simulink model "No6_QuadcopterTrackPositionControl"  (R2022a)
settings: Solver=FixedStepDiscrete  StartTime=0.0  StopTime=Inf  RelTol=1e-3  EnableMultiTasking=on
undefined symbols (not defined in the file): dev, DiscIntNeverNeededParam, Main, pwm_output0
libraries: slpidlib x7, simulink x1, px4lib x1, px4uORBlib x1, sharedtransform x1
settings Model: PacingRate=1000  ExtModeTrigDuration=10  Creator=liuwhale  LastModifiedBy=liuwhale
settings SolverCC: PositivePriorityOrder=on
settings DataIOCC: ReturnWorkspaceOutputsName=tp3ab4fdac_68ba_4606_82f6_9556b5dbcc17
settings OptimizationCC: EnhancedBackFolding=on  PassReuseOutputArgsAs=Individual arguments  ZeroExternalMemoryAtStartup=off  ZeroInternalMemoryAtStartup=off  MaxStackSize=64  OptimizeBlockOrder=speed  DifferentSizesBufferReuse=on  EfficientTunableParamExpr=on
settings DebuggingCC: ParameterTunabilityLossMsg=error
settings HardwareCC: ProdBitPerPointer=32  ProdBitPerSizeT=32  ProdBitPerPtrDiffT=32  ProdLargestAtomicInteger=Long  ProdLargestAtomicFloat=Double  ProdWordSize=32  ProdLongLongMode=on  ProdHWDeviceType=ARM Compatible->ARM Cortex
settings SFSimCC: MATLABDynamicMemAlloc=off  SimTargetLang=C++
settings RTWCC: SystemTargetFile=ert.tlc  HardwareBoard=PX4 Host Target  TLCOptions="-aInlineSetEventsForThisBaseRateFcn=TLC_FALSE -aSuppressMultiTaskScheduler=TLC_FALSE  -aRateBasedStepFcn=0"  TemplateMakefile=ert_default_tmf  Toolchain=GNU Tools for PX4 Autopilots  PortableWordSizes=on  TargetLang=C++
settings CodeAppCC: ForceParamTrailComments=on  IgnoreCustomStorageClasses=off  OperatorAnnotations=on  SimulinkDataObjDesc=on  SFDataObjDesc=on  InsertBlockDesc=on
settings ERTTargetCC: ExtModeStaticAlloc=on

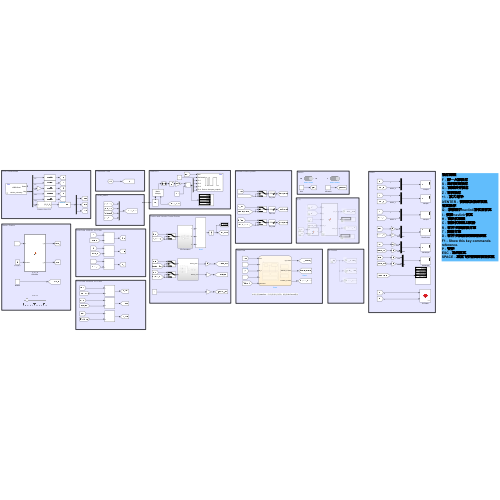
[thumbnail: Simulink's stored preview of the top-level diagram]
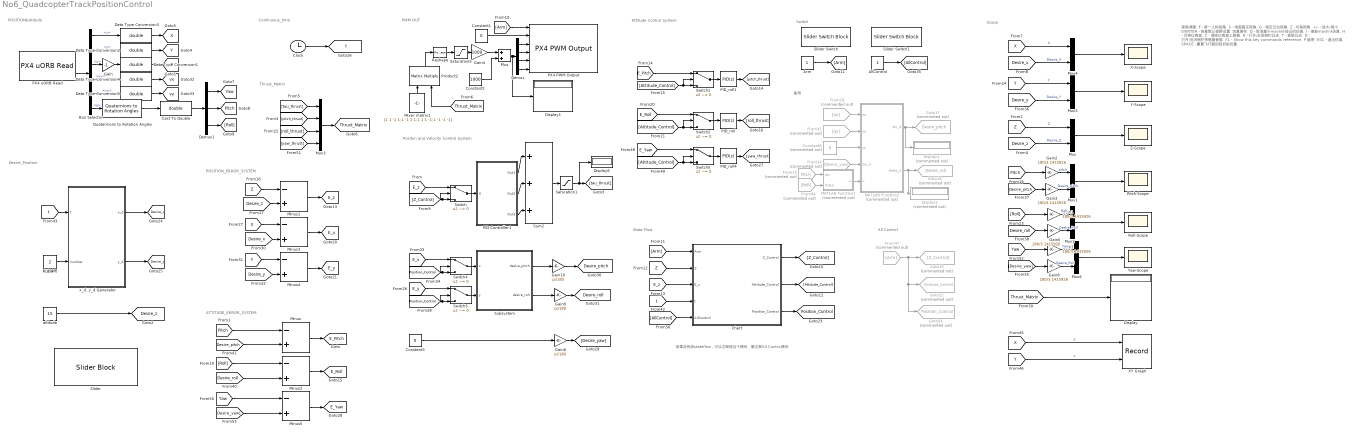
== system No6_QuadcopterTrackPositionControl ==
  note: 如果没有装stateflow，可以注释掉这个模块，解注释All Control模块
  note: All Control
  note: Desire_Position
  note: 备用
  note: 视角调整:
      | F - 第一人称视角.
      | S - 地面固定视角.
      | G - 稳定云台视角.
      | Z - 切换视角.
      | +/- - 放大/缩小
      | 0/ENTER - 恢复默认视野设置.
      | 仿真操作:
      | Q - 取消基于mavlink协议的仿真.
      | I - 使能mavlink仿真.
      | H - 切换仪表盘.
      | C - 清除仪表盘上数据.
      | R - 打开/关闭侧栏日志.
      | T - 更新日志.
      | D - 打开/关闭侧栏传感器参数.
      | F1 - Show this key commands reference.
      | P - 暂停.
      | ESC - 退出仿真.
      | SPACE - 重置飞行器回到初始位置.
  note: State Flow
  note: PWM OUT
  note: Scope
  note: Positon and Velocity Control System
  note: Thrust_Matrix
  note: POSITION_ERROR_SYSTEM
  note: POSITION&Atitude
  note: Continuous_time
  note: Switch
  note: Attitude Control System
  note: ATTITUDE_ERROR_SYSTEM
  AllControl : Constant  OutDataTypeStr=boolean
  Arm : Constant  OutDataTypeStr=boolean
  Bus Selector : BusSelector  OutputSignals=x,y,z,vx,vy,q
  Cast To Double : DataTypeConversion  OutDataTypeStr=double  SaturateOnIntegerOverflow=off  RndMeth=Floor
  Chart : Stateflow chart  TreatAsAtomicUnit=on
  Clock : Clock
  Constant1 : Constant  Value=0  OutDataTypeStr=boolean
  Constant2 : Constant  Value=1000  OutDataTypeStr=uint16
  Constant3 : Constant  Value=0
  Constant6 : Constant  Commented=on  Value=0
  Data Type Conversion{1..5} (5 alike) : DataTypeConversion  OutDataTypeStr=double  SaturateOnIntegerOverflow=off  RndMeth=Floor
  Demux : Demux
  Demux1 : Demux  Outputs=3
  Display : Display
  Display1 : Display
  Display4 : Display  Commented=on
  Display5 : Display  Commented=on
  Display6 : Display
  From25 : From  Commented=on  GotoTag=Pitch  TagVisibility=global
  From29 : From  Commented=on  GotoTag=qx
  From35 : From  Commented=on  GotoTag=qy
  From44 : From  Commented=on  GotoTag=Roll
  From47 : From  Commented=on  GotoTag=Arm
  From54 : From  Commented=on  GotoTag=Desire_yaw
  Gain : Gain  Gain=-1
  Gain{1..3,5,7..8} (6 alike) : Gain  Gain=180/3.1415926
  Gain10 : Gain  Gain=pi/180
  Gain4 : Gain  Gain=1000  OutDataTypeStr=uint16
  Gain6 : Gain  Gain=pi/180
  Gain9 : Gain  Gain=pi/180
  Goto17 : Goto  Commented=on  GotoTag=Desire_pitch  TagVisibility=global
  Goto18 : Goto  Commented=on  GotoTag=Desire_roll  TagVisibility=global
  Goto19 : Goto  Commented=on  GotoTag=Z_Control
  Goto22 : Goto  Commented=on  GotoTag=Attitude_Control
  Goto34 : Goto  Commented=on  GotoTag=Position_Control  TagVisibility=global
  MATLAB Function1 : MATLAB Function  Commented=on  TreatAsAtomicUnit=on
  MATLAB Function2 : MATLAB Function  Commented=on  TreatAsAtomicUnit=on
  Minus{,1..5} (6 alike) : Sum  Inputs=-+
  Mixer matrix1 : Constant  Value=[1 1 -1 1;1 -1 1 1;1 1 1 -1;1 -1 -1 -1]  OutDataTypeStr=Inherit: Inherit via back propagation
  Mux{,1..2,4..6} (6 alike) : Mux  Inputs=2
  Mux3 : Mux
  PID Controller1 : Subsystem
  PID_roll : slpidlib/PID Controller  Controller=PID  Form=Parallel  TimeDomain=Discrete-time  UseExternalTs=off  SampleTime=-1  IntegratorMethod=Backward Euler  FilterMethod=Forward Euler  ControllerParametersSource=internal  P=0.038  I=0.06  UseKiTs=off  D=0.001  N=100  UseFilter=on  TunerSelectOption=Transfer Function Based (PID Tuner App)  InitialConditionSource=internal  InitialConditionForIntegrator=0  InitialConditionForFilter=0  DifferentiatorICPrevScaledInput=0  ExternalReset=none  TrackingMode=off  Kt=1  LimitOutput=on  SatLimitsSource=internal  UpperSaturationLimit=0.01  LowerSaturationLimit=-0.01  LinearizeAsGain=off  AntiWindupMode=none  Kb=1  POutMin=[]  POutMax=[]  IOutMin=[]  IOutMax=[]  DOutMin=[]  DOutMax=[]  NOutMin=[]  NOutMax=[]  SumOutMin=[]  SumOutMax=[]  SaturationOutMin=[]  SaturationOutMax=[]  PParamMin=[]  PParamMax=[]  IParamMin=[]  IParamMax=[]  DParamMin=[]  DParamMax=[]  NParamMin=[]  NParamMax=[]  KbParamMin=[]  KbParamMax=[]  KtParamMin=[]  KtParamMax=[]  KbOutMin=[]  KbOutMax=[]  KtOutMin=[]  KtOutMax=[]  IntegratorOutMin=[]  IntegratorOutMax=[]  FilterOutMin=[]  FilterOutMax=[]  SumI1OutMin=[]  SumI1OutMax=[]  SumI2OutMin=[]  SumI2OutMax=[]  SumI3OutMin=[]  SumI3OutMax=[]  SumI4OutMin=[]  SumI4OutMax=[]  SumDOutMin=[]  SumDOutMax=[]  DifferentiatorOutMin=[]  DifferentiatorOutMax=[]  FilterDiffOutCoefMin=[]  FilterDiffOutCoefMax=[]  ReciprocalOutMin=[]  ReciprocalOutMax=[]  SumDenOutMin=[]  SumDenOutMax=[]  SumNumOutMin=[]  SumNumOutMax=[]  DivideOutMin=[]  DivideOutMax=[]  UdiffTsProdOutMin=[]  UdiffTsProdOutMax=[]  NTsProdOutMin=[]  NTsProdOutMax=[]  UintegralTsProdOutMin=[]  UintegralTsProdOutMax=[]  UngainTsProdOutMin=[]  UngainTsProdOutMax=[]  IntegratorContinuousStateAttributes=''  IntegratorStateMustResolveToSignalObject=off  IntegratorRTWStateStorageClass=Auto  FilterContinuousStateAttributes=''  FilterStateMustResolveToSignalObject=off  FilterRTWStateStorageClass=Auto  ParallelPVariant=InternalParameters  IdealPVariant=Disabled  IVariant=InternalParameters  DVariant=InternalParameters  IntegratorVariant=Discrete  SatVariant=Enabled  AWVariant=Passthrough  PCopyVariant=Disabled  TRVariant=Disabled  FdbkBlocksVariant=Forward  IdealPFdbkVariant=Disabled  SatFdbkVariant=Disabled  DerivativeFilterVariant=ForwardEulerFilter  NVariant=InternalParameters  NCopyVariant=Disabled  FilterICVariant=InternalICsFilter  IntegratorICVariant=InternalICs  ExternalResetVariant=Disabled  TRSumVariant=Passthrough  SumFdbkVariant=Disabled  SumVariant=Sum_PID  TsampFilterVariant=InternalTs  TsampNgainVariant=Passthrough  TsampIntegralVariant=Passthrough  ExternalSaturationOutDataTypeStr=Inherit: Same as second input  aMode=0
  PID_roll1 : slpidlib/PID Controller  Controller=PID  Form=Parallel  TimeDomain=Discrete-time  UseExternalTs=off  SampleTime=-1  IntegratorMethod=Backward Euler  FilterMethod=Forward Euler  ControllerParametersSource=internal  P=0.038  I=0.06  UseKiTs=off  D=0.001  N=100  UseFilter=on  TunerSelectOption=Transfer Function Based (PID Tuner App)  InitialConditionSource=internal  InitialConditionForIntegrator=0  InitialConditionForFilter=0  DifferentiatorICPrevScaledInput=0  ExternalReset=none  TrackingMode=off  Kt=1  LimitOutput=on  SatLimitsSource=internal  UpperSaturationLimit=0.01  LowerSaturationLimit=-0.01  LinearizeAsGain=off  AntiWindupMode=none  Kb=1  POutMin=[]  POutMax=[]  IOutMin=[]  IOutMax=[]  DOutMin=[]  DOutMax=[]  NOutMin=[]  NOutMax=[]  SumOutMin=[]  SumOutMax=[]  SaturationOutMin=[]  SaturationOutMax=[]  PParamMin=[]  PParamMax=[]  IParamMin=[]  IParamMax=[]  DParamMin=[]  DParamMax=[]  NParamMin=[]  NParamMax=[]  KbParamMin=[]  KbParamMax=[]  KtParamMin=[]  KtParamMax=[]  KbOutMin=[]  KbOutMax=[]  KtOutMin=[]  KtOutMax=[]  IntegratorOutMin=[]  IntegratorOutMax=[]  FilterOutMin=[]  FilterOutMax=[]  SumI1OutMin=[]  SumI1OutMax=[]  SumI2OutMin=[]  SumI2OutMax=[]  SumI3OutMin=[]  SumI3OutMax=[]  SumI4OutMin=[]  SumI4OutMax=[]  SumDOutMin=[]  SumDOutMax=[]  DifferentiatorOutMin=[]  DifferentiatorOutMax=[]  FilterDiffOutCoefMin=[]  FilterDiffOutCoefMax=[]  ReciprocalOutMin=[]  ReciprocalOutMax=[]  SumDenOutMin=[]  SumDenOutMax=[]  SumNumOutMin=[]  SumNumOutMax=[]  DivideOutMin=[]  DivideOutMax=[]  UdiffTsProdOutMin=[]  UdiffTsProdOutMax=[]  NTsProdOutMin=[]  NTsProdOutMax=[]  UintegralTsProdOutMin=[]  UintegralTsProdOutMax=[]  UngainTsProdOutMin=[]  UngainTsProdOutMax=[]  IntegratorContinuousStateAttributes=''  IntegratorStateMustResolveToSignalObject=off  IntegratorRTWStateStorageClass=Auto  FilterContinuousStateAttributes=''  FilterStateMustResolveToSignalObject=off  FilterRTWStateStorageClass=Auto  ParallelPVariant=InternalParameters  IdealPVariant=Disabled  IVariant=InternalParameters  DVariant=InternalParameters  IntegratorVariant=Discrete  SatVariant=Enabled  AWVariant=Passthrough  PCopyVariant=Disabled  TRVariant=Disabled  FdbkBlocksVariant=Forward  IdealPFdbkVariant=Disabled  SatFdbkVariant=Disabled  DerivativeFilterVariant=ForwardEulerFilter  NVariant=InternalParameters  NCopyVariant=Disabled  FilterICVariant=InternalICsFilter  IntegratorICVariant=InternalICs  ExternalResetVariant=Disabled  TRSumVariant=Passthrough  SumFdbkVariant=Disabled  SumVariant=Sum_PID  TsampFilterVariant=InternalTs  TsampNgainVariant=Passthrough  TsampIntegralVariant=Passthrough  ExternalSaturationOutDataTypeStr=Inherit: Same as second input  aMode=0
  PID_roll4 : slpidlib/PID Controller  Controller=PID  Form=Parallel  TimeDomain=Discrete-time  UseExternalTs=off  SampleTime=-1  IntegratorMethod=Backward Euler  FilterMethod=Forward Euler  ControllerParametersSource=internal  P=0.055  I=0.05  UseKiTs=off  D=0.003  N=100  UseFilter=on  TunerSelectOption=Transfer Function Based (PID Tuner App)  InitialConditionSource=internal  InitialConditionForIntegrator=0  InitialConditionForFilter=0  DifferentiatorICPrevScaledInput=0  ExternalReset=none  TrackingMode=off  Kt=1  LimitOutput=on  SatLimitsSource=internal  UpperSaturationLimit=0.01  LowerSaturationLimit=-0.01  LinearizeAsGain=off  AntiWindupMode=none  Kb=1  POutMin=[]  POutMax=[]  IOutMin=[]  IOutMax=[]  DOutMin=[]  DOutMax=[]  NOutMin=[]  NOutMax=[]  SumOutMin=[]  SumOutMax=[]  SaturationOutMin=[]  SaturationOutMax=[]  PParamMin=[]  PParamMax=[]  IParamMin=[]  IParamMax=[]  DParamMin=[]  DParamMax=[]  NParamMin=[]  NParamMax=[]  KbParamMin=[]  KbParamMax=[]  KtParamMin=[]  KtParamMax=[]  KbOutMin=[]  KbOutMax=[]  KtOutMin=[]  KtOutMax=[]  IntegratorOutMin=[]  IntegratorOutMax=[]  FilterOutMin=[]  FilterOutMax=[]  SumI1OutMin=[]  SumI1OutMax=[]  SumI2OutMin=[]  SumI2OutMax=[]  SumI3OutMin=[]  SumI3OutMax=[]  SumI4OutMin=[]  SumI4OutMax=[]  SumDOutMin=[]  SumDOutMax=[]  DifferentiatorOutMin=[]  DifferentiatorOutMax=[]  FilterDiffOutCoefMin=[]  FilterDiffOutCoefMax=[]  ReciprocalOutMin=[]  ReciprocalOutMax=[]  SumDenOutMin=[]  SumDenOutMax=[]  SumNumOutMin=[]  SumNumOutMax=[]  DivideOutMin=[]  DivideOutMax=[]  UdiffTsProdOutMin=[]  UdiffTsProdOutMax=[]  NTsProdOutMin=[]  NTsProdOutMax=[]  UintegralTsProdOutMin=[]  UintegralTsProdOutMax=[]  UngainTsProdOutMin=[]  UngainTsProdOutMax=[]  IntegratorContinuousStateAttributes=''  IntegratorStateMustResolveToSignalObject=off  IntegratorRTWStateStorageClass=Auto  FilterContinuousStateAttributes=''  FilterStateMustResolveToSignalObject=off  FilterRTWStateStorageClass=Auto  ParallelPVariant=InternalParameters  IdealPVariant=Disabled  IVariant=InternalParameters  DVariant=InternalParameters  IntegratorVariant=Discrete  SatVariant=Enabled  AWVariant=Passthrough  PCopyVariant=Disabled  TRVariant=Disabled  FdbkBlocksVariant=Forward  IdealPFdbkVariant=Disabled  SatFdbkVariant=Disabled  DerivativeFilterVariant=ForwardEulerFilter  NVariant=InternalParameters  NCopyVariant=Disabled  FilterICVariant=InternalICsFilter  IntegratorICVariant=InternalICs  ExternalResetVariant=Disabled  TRSumVariant=Passthrough  SumFdbkVariant=Disabled  SumVariant=Sum_PID  TsampFilterVariant=InternalTs  TsampNgainVariant=Passthrough  TsampIntegralVariant=Passthrough  ExternalSaturationOutDataTypeStr=Inherit: Same as second input  aMode=0
  PX4 PWM Output : px4lib/PX4 PWM Output  pwmDevice=Main (/dev/pwm_output0)  pwmChannel1_=on  pwmChannel2_=on  pwmChannel3_=on  pwmChannel4_=on  pwmChannel5_=off  pwmChannel6_=off  pwmChannel7_=off  pwmChannel8_=off  forceTerminateFailsafe=off  outputErrorStatus=off
      settings: SourceProductBaseCode=PX4AUTOPILOTS
  PX4 uORB Read : px4uORBlib/PX4 uORB Read  uORBTopic=vehicle_odometry  selectInstance=vehicle_odometry  SampleTime=0.001  BlockingMode=off  BlockTimeout=1e-3
      settings: SourceProductBaseCode=PX4AUTOPILOTS
  Pitch-Scope : Scope
  Plus : Sum
  Product2 : Product  Multiplication=Matrix(*)  RndMeth=Zero
  Quaternions to Rotation Angles : sharedtransform/Quaternions to Rotation Angles  rotationOrder=ZYX  aMode=aMode
      settings: SourceProductBaseCode=AE,PW,DR,MT,VE
  Reshape : Reshape  OutputDimensionality=Row vector (2-D)
  Roll-Scope : Scope
  Saturation1 : Saturate  UpperLimit=1.6  LowerLimit=-1.6
  Saturation5 : Saturate  UpperLimit=1  LowerLimit=0
  Slider : SliderBlock
  Slider Switch : SliderSwitchBlock
      settings: Values={{'Off', 'On'}, [0 1]}
  Slider Switch1 : SliderSwitchBlock
      settings: Values={{'Off', 'On'}, [0 1]}
  Subsystem : Subsystem
  Sum2 : Sum  Inputs=|+++
  Switch{,1..5} (6 alike) : Switch  Criteria=u2 ~= 0  SaturateOnIntegerOverflow=off  InputSameDT=off
  X-Scope : Scope
  XY Graph : Record  FileSettingsInternal="{\"entries\":[{\"content\":{\"excelSettings\":{\"content\":{},\"type\":\"Streamout.ExcelSettings\"}},\"type\":\"Streamout.FileSettingStorage\",\"uuid\":\"24123f32-9ba5-4678-86a6-e7377285f4b6\"}],\"packageUris\":[\"http://schema.mathworks.com/mf0/streamout_blocks/R2020a\"],\"version\":\"1.0\"}"  Layout=[1 1]  SignalsInternal="{\"entries\":[{\"content\":{\"signals\":[{\"content\":{\"blockPath\":[\"No6_QuadcopterAtitudeControl/XY Graph\"],\"channel\":[],\"dimensions\":[1,1],\"domain\":\"No6_QuadcopterAtitudeControl/XY Graph\",\"lineColor\":\"#a2142f\",\"plots\":[1],\"port\":1,\"sid\":[\"\"],\"signalID\":152052,\"signalName\":\"X\"},\"type\":\"RecordBlkView.Signal\",\"uuid\":\"5969967d-d21d-4a5b-9289-edafa093ff5a\"},{\"content\":{\"blockPath\":[\"No6_QuadcopterAtitudeControl/XY Graph\"],\"channel\":[],\"dimensions\":[1,1],\"domain\":\"No6_QuadcopterAtitudeControl/XY Graph\",\"lineColor\":\"#139fff\",\"plots\":[1],\"port\":2,\"sid\":[\"\"],\"signalID\":152056,\"signalName\":\"Y\"},\"type\":\"RecordBlkView.Signal\",\"uuid\":\"db06691f-44cf-4505-9bbe-a7e47946ba1d\"}]},\"type\":\"RecordBlkView.InputSignals\",\"uuid\":\"46524bf0-71bf-4488-84ce-6e309663723d\"}],\"packageUris\":[\"http://schema.mathworks.com/mf0/streamout_blocks/R2020a\"],\"version\":\"1.0\"}"  VisualizationBindings="{\"xyplotplugin\":{\"info\":[{\"series\":[{\"bindingParametersList\":[{\"parameter\":\"X-Axis\",\"signalID\":152052,\"signalName\":\"X\"},{\"parameter\":\"Y-Axis\",\"signalID\":152056,\"signalName\":\"Y\"}],\"seriesID\":212}],\"subplotID\":1}]}}"  CompatibilityTag=XY
  Y-Scope : Scope
  Yaw-Scope : Scope
  Z-Scope : Scope
  altitude : Constant  Value=15
  "x_d, y_d Generator" : MATLAB Function  TreatAsAtomicUnit=on
  轨迹编号 : Constant  Value=2
  tag scope: Desire_pitch=global, Desire_roll=global, Desire_x=global, Desire_y=global, Desire_z=global, E_Pitch=global, E_Roll=global, E_Yaw=global, E_x=global, E_y=global, E_z=global, Pitch=global, Position_Control=global, Thrust_Matrix=global, X=global, Y=global, Yaw=global, Z=global, t=global, vx=global, vy=global
  wires:
  [Arm] -> PX4 PWM Output/1
  Constant1/1 -> PX4 PWM Output/2
  Mixer matrix1/1 -> Product2/1
  Demux/1 -> PX4 PWM Output/3
  Demux/2 -> PX4 PWM Output/4
  Demux/3 -> PX4 PWM Output/5
  Demux/4 -> PX4 PWM Output/6
  Minus/1 -> [E_Pitch]
  Bus Selector/3 -> Gain/1  "<z>"
  PX4 uORB Read/2 -> Bus Selector/1
  Gain/1 -> Data Type Conversion1/1
  Mux/1 -> Z-Scope/1
  [Z] -> Mux/1  "Z"
  [Desire_z] -> Mux/2  "Desire_Z"
  [Pitch] -> Minus/1
  Data Type Conversion1/1 -> [Z]
  altitude/1 -> [Desire_z]
  [E_z] -> Switch/1
  [tau_thrust] -> Mux3/1
  Mux3/1 -> [Thrust_Matrix]
  Data Type Conversion2/1 -> [Y]
  Bus Selector/2 -> Data Type Conversion2/1  "<y>"
  Data Type Conversion3/1 -> [X]
  Bus Selector/1 -> Data Type Conversion3/1  "<x>"
  [Thrust_Matrix] -> Product2/2
  [Z_Control] -> Switch/2, Switch/3
  Sum2/1 -> Saturation1/1
  Demux1/2 -> [Pitch]
  Quaternions to Rotation Angles/1 -> Cast To Double/1
  Cast To Double/1 -> Demux1/1
  Demux1/3 -> [Roll]
  Demux1/1 -> [Yaw]
  Bus Selector/6 -> Quaternions to Rotation Angles/1  "<q>"
  [Arm] -> Chart/1(Arm)
  Arm/1 -> [Arm]
  [Z] -> Chart/2(Z)
  [E_z] -> Chart/3(E_z)
  [Attitude_Control] -> Switch1/3, Switch1/2
  Switch1/1 -> PID_roll1/1
  [E_Pitch] -> Switch1/1
  [Z] -> Minus1/1
  Minus1/1 -> [E_z]
  [pitch_thrust] -> Mux3/2
  [Desire_pitch] -> Gain3/1
  [Pitch] -> Gain2/1
  Minus2/1 -> [E_Roll]
  Switch2/1 -> PID_roll/1
  [E_Roll] -> Switch2/1
  [Attitude_Control] -> Switch2/3, Switch2/2
  [Roll] -> Minus2/1
  [Desire_roll] -> Gain5/1
  [Roll] -> Gain1/1
  "x_d, y_d Generator"/1(x_d) -> [Desire_x]
  [t] -> "x_d, y_d Generator"/1(t)
  "x_d, y_d Generator"/2(y_d) -> [Desire_y]
  MATLAB Function1/1(u) -> MATLAB Function2/5(u)
  Constant6/1 -> MATLAB Function2/3(qz)
  [Position_Control] -> Switch3/2, Switch3/3
  Minus3/1 -> [E_x]
  [X] -> Minus3/1
  [Y] -> Minus4/1
  Minus4/1 -> [E_y]
  [Position_Control] -> Switch4/2, Switch4/3
  [Desire_x] -> Mux4/2  "Desire_X"
  [X] -> Mux4/1  "X"
  Mux4/1 -> X-Scope/1
  Mux5/1 -> Y-Scope/1
  [Y] -> Mux5/1  "Y"
  [Desire_y] -> Mux5/2  "Desire_Y"
  [Thrust_Matrix] -> Display/1
  PID_roll/1 -> [roll_thrust]
  PID_roll1/1 -> [pitch_thrust]
  [E_y] -> Switch3/1
  [E_x] -> Switch4/1
  Mux2/1 -> Roll-Scope/1
  Mux1/1 -> Pitch-Scope/1
  Gain2/1 -> Mux1/1  "pitch"
  Gain3/1 -> Mux1/2  "Desire_pitch"
  Gain1/1 -> Mux2/1  "Roll"
  Gain5/1 -> Mux2/2  "Desire_Roll"
  [X] -> XY Graph/1  "X"
  [Y] -> XY Graph/2  "Y"
  [Desire_roll] -> Minus2/2
  [Desire_z] -> Minus1/2
  [Desire_y] -> Minus4/2
  [Desire_x] -> Minus3/2
  [Desire_pitch] -> Minus/2
  Plus/1 -> Display1/1, Demux/1
  Gain4/1 -> Plus/1
  Constant2/1 -> Plus/2
  Reshape/1 -> Saturation5/1
  Saturation5/1 -> Gain4/1
  Product2/1 -> Reshape/1
  PID Controller1/2(Out2) -> Sum2/2
  PID Controller1/3(Out3) -> Sum2/3
  PID Controller1/1(Out1) -> Sum2/1
  Switch/1 -> PID Controller1/1(U)
  Saturation1/1 -> Display6/1, [tau_thrust]
  Clock/1 -> [t]
  [t] -> Chart/4(t)
  MATLAB Function2/2(theta_d) -> Goto18/1, Display5/1
  From29/1 -> MATLAB Function2/1(qx)
  From35/1 -> MATLAB Function2/2(qy)
  From25/1 -> MATLAB Function1/1(phi)
  From44/1 -> MATLAB Function1/2(theta)
  [roll_thrust] -> Mux3/3
  PID_roll4/1 -> [yaw_thrust]
  [E_Yaw] -> Switch5/1
  [Attitude_Control] -> Switch5/3, Switch5/2
  Switch5/1 -> PID_roll4/1
  [Yaw] -> Minus5/1
  Minus5/1 -> [E_Yaw]
  [yaw_thrust] -> Mux3/4
  [Yaw] -> Gain7/1
  [Desire_yaw] -> Minus5/2
  Constant3/1 -> Gain6/1
  Gain6/1 -> [Desire_yaw]
  From54/1 -> MATLAB Function2/4(psi_d)
  Mux6/1 -> Yaw-Scope/1
  Gain7/1 -> Mux6/1  "Yaw"
  [Desire_yaw] -> Gain8/1
  Gain8/1 -> Mux6/2  "Desire_Roll"
  MATLAB Function2/1(phi_d) -> Goto17/1, Display4/1
  Gain9/1 -> [Desire_roll]
  Gain10/1 -> [Desire_pitch]
  Subsystem/2(desire_roll) -> Gain9/1
  Subsystem/1(desire_pitch) -> Gain10/1
  Switch4/1 -> Subsystem/1(x)
  Bus Selector/4 -> Data Type Conversion4/1  "<vx>"
  Data Type Conversion4/1 -> [vx]
  Data Type Conversion5/1 -> [vy]
  Bus Selector/5 -> Data Type Conversion5/1  "<vy>"
  Switch3/1 -> Subsystem/2(y)
  轨迹编号/1 -> "x_d, y_d Generator"/2(number)
  Chart/2(Attitude_Control) -> [Attitude_Control]
  Chart/1(Z_Control) -> [Z_Control]
  Chart/3(Position_Control) -> [Position_Control]
  From47/1 -> Goto34/1, Goto22/1, Goto19/1
  AllControl/1 -> [AllControl]
  [AllControl] -> Chart/5(AllControl)

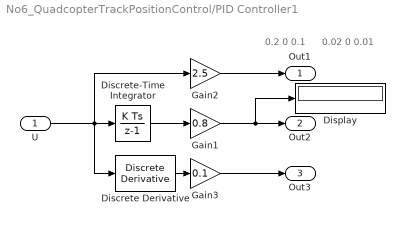
== system No6_QuadcopterTrackPositionControl/PID Controller1 ==
  note: 0.2 0 0.1
  note: 0.02 0 0.01
  U : Inport
  Discrete Derivative : simulink/Discrete/Discrete Derivative  gainval=1.0  ICPrevScaledInput=0.0  OutMin=[]  OutMax=[]  OutDataType=fixdt(1, 16)  OutScaling=2^-10  DoSatur=off
  Discrete-Time Integrator : DiscreteIntegrator  SampleTime=-1  UpperSaturationLimit=1.7  LowerSaturationLimit=-1.7  ICPrevOutput=DiscIntNeverNeededParam  ICPrevScaledInput=DiscIntNeverNeededParam
  Display : Display
  Gain1 : Gain  Gain=0.8
  Gain2 : Gain  Gain=2.5
  Gain3 : Gain  Gain=0.1
  Out1 : Outport
  Out2 : Outport  Port=2
  Out3 : Outport  Port=3
  wires:
  Discrete Derivative/1 -> Gain3/1
  U/1 -> Gain2/1, Discrete Derivative/1, Discrete-Time Integrator/1
  Gain3/1 -> Out3/1
  Gain1/1 -> Display/1, Out2/1
  Discrete-Time Integrator/1 -> Gain1/1
  Gain2/1 -> Out1/1

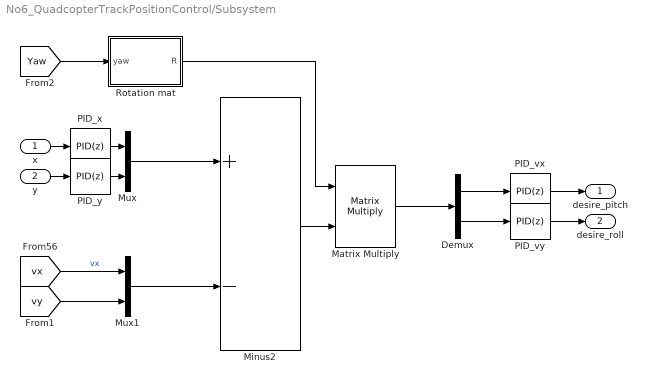
== system No6_QuadcopterTrackPositionControl/Subsystem ==
  x : Inport
  y : Inport  Port=2
  Demux : Demux  Outputs=2
  Matrix Multiply : Product  Multiplication=Matrix(*)
  Minus2 : Sum  Inputs=+-
  Mux : Mux  Inputs=2
  Mux1 : Mux  Inputs=2
  PID_vx : slpidlib/PID Controller  Controller=PID  Form=Parallel  TimeDomain=Discrete-time  UseExternalTs=off  SampleTime=-1  IntegratorMethod=Forward Euler  FilterMethod=Forward Euler  ControllerParametersSource=internal  P=4  I=0.01  UseKiTs=off  D=1  N=1  UseFilter=on  TunerSelectOption=Transfer Function Based (PID Tuner App)  InitialConditionSource=internal  InitialConditionForIntegrator=0  InitialConditionForFilter=0  DifferentiatorICPrevScaledInput=0  ExternalReset=none  TrackingMode=off  Kt=1  LimitOutput=on  SatLimitsSource=internal  UpperSaturationLimit=30  LowerSaturationLimit=-30  LinearizeAsGain=off  AntiWindupMode=none  Kb=1  POutMin=[]  POutMax=[]  IOutMin=[]  IOutMax=[]  DOutMin=[]  DOutMax=[]  NOutMin=[]  NOutMax=[]  SumOutMin=[]  SumOutMax=[]  SaturationOutMin=[]  SaturationOutMax=[]  PParamMin=[]  PParamMax=[]  IParamMin=[]  IParamMax=[]  DParamMin=[]  DParamMax=[]  NParamMin=[]  NParamMax=[]  KbParamMin=[]  KbParamMax=[]  KtParamMin=[]  KtParamMax=[]  KbOutMin=[]  KbOutMax=[]  KtOutMin=[]  KtOutMax=[]  IntegratorOutMin=[]  IntegratorOutMax=[]  FilterOutMin=[]  FilterOutMax=[]  SumI1OutMin=[]  SumI1OutMax=[]  SumI2OutMin=[]  SumI2OutMax=[]  SumI3OutMin=[]  SumI3OutMax=[]  SumI4OutMin=[]  SumI4OutMax=[]  SumDOutMin=[]  SumDOutMax=[]  DifferentiatorOutMin=[]  DifferentiatorOutMax=[]  FilterDiffOutCoefMin=[]  FilterDiffOutCoefMax=[]  ReciprocalOutMin=[]  ReciprocalOutMax=[]  SumDenOutMin=[]  SumDenOutMax=[]  SumNumOutMin=[]  SumNumOutMax=[]  DivideOutMin=[]  DivideOutMax=[]  UdiffTsProdOutMin=[]  UdiffTsProdOutMax=[]  NTsProdOutMin=[]  NTsProdOutMax=[]  UintegralTsProdOutMin=[]  UintegralTsProdOutMax=[]  UngainTsProdOutMin=[]  UngainTsProdOutMax=[]  IntegratorContinuousStateAttributes=''  IntegratorStateMustResolveToSignalObject=off  IntegratorRTWStateStorageClass=Auto  FilterContinuousStateAttributes=''  FilterStateMustResolveToSignalObject=off  FilterRTWStateStorageClass=Auto  ParallelPVariant=InternalParameters  IdealPVariant=Disabled  IVariant=InternalParameters  DVariant=InternalParameters  IntegratorVariant=Discrete  SatVariant=Enabled  AWVariant=Passthrough  PCopyVariant=Disabled  TRVariant=Disabled  FdbkBlocksVariant=Forward  IdealPFdbkVariant=Disabled  SatFdbkVariant=Disabled  DerivativeFilterVariant=ForwardEulerFilter  NVariant=InternalParameters  NCopyVariant=Disabled  FilterICVariant=InternalICsFilter  IntegratorICVariant=InternalICs  ExternalResetVariant=Disabled  TRSumVariant=Passthrough  SumFdbkVariant=Disabled  SumVariant=Sum_PID  TsampFilterVariant=InternalTs  TsampNgainVariant=Passthrough  TsampIntegralVariant=Passthrough  ExternalSaturationOutDataTypeStr=Inherit: Same as second input  aMode=0
  PID_vy : slpidlib/PID Controller  Controller=PID  Form=Parallel  TimeDomain=Discrete-time  UseExternalTs=off  SampleTime=-1  IntegratorMethod=Backward Euler  FilterMethod=Forward Euler  ControllerParametersSource=internal  P=4  I=0.01  UseKiTs=off  D=1  N=1  UseFilter=on  TunerSelectOption=Transfer Function Based (PID Tuner App)  InitialConditionSource=internal  InitialConditionForIntegrator=0  InitialConditionForFilter=0  DifferentiatorICPrevScaledInput=0  ExternalReset=none  TrackingMode=off  Kt=1  LimitOutput=on  SatLimitsSource=internal  UpperSaturationLimit=30  LowerSaturationLimit=-30  LinearizeAsGain=off  AntiWindupMode=none  Kb=1  POutMin=[]  POutMax=[]  IOutMin=[]  IOutMax=[]  DOutMin=[]  DOutMax=[]  NOutMin=[]  NOutMax=[]  SumOutMin=[]  SumOutMax=[]  SaturationOutMin=[]  SaturationOutMax=[]  PParamMin=[]  PParamMax=[]  IParamMin=[]  IParamMax=[]  DParamMin=[]  DParamMax=[]  NParamMin=[]  NParamMax=[]  KbParamMin=[]  KbParamMax=[]  KtParamMin=[]  KtParamMax=[]  KbOutMin=[]  KbOutMax=[]  KtOutMin=[]  KtOutMax=[]  IntegratorOutMin=[]  IntegratorOutMax=[]  FilterOutMin=[]  FilterOutMax=[]  SumI1OutMin=[]  SumI1OutMax=[]  SumI2OutMin=[]  SumI2OutMax=[]  SumI3OutMin=[]  SumI3OutMax=[]  SumI4OutMin=[]  SumI4OutMax=[]  SumDOutMin=[]  SumDOutMax=[]  DifferentiatorOutMin=[]  DifferentiatorOutMax=[]  FilterDiffOutCoefMin=[]  FilterDiffOutCoefMax=[]  ReciprocalOutMin=[]  ReciprocalOutMax=[]  SumDenOutMin=[]  SumDenOutMax=[]  SumNumOutMin=[]  SumNumOutMax=[]  DivideOutMin=[]  DivideOutMax=[]  UdiffTsProdOutMin=[]  UdiffTsProdOutMax=[]  NTsProdOutMin=[]  NTsProdOutMax=[]  UintegralTsProdOutMin=[]  UintegralTsProdOutMax=[]  UngainTsProdOutMin=[]  UngainTsProdOutMax=[]  IntegratorContinuousStateAttributes=''  IntegratorStateMustResolveToSignalObject=off  IntegratorRTWStateStorageClass=Auto  FilterContinuousStateAttributes=''  FilterStateMustResolveToSignalObject=off  FilterRTWStateStorageClass=Auto  ParallelPVariant=InternalParameters  IdealPVariant=Disabled  IVariant=InternalParameters  DVariant=InternalParameters  IntegratorVariant=Discrete  SatVariant=Enabled  AWVariant=Passthrough  PCopyVariant=Disabled  TRVariant=Disabled  FdbkBlocksVariant=Forward  IdealPFdbkVariant=Disabled  SatFdbkVariant=Disabled  DerivativeFilterVariant=ForwardEulerFilter  NVariant=InternalParameters  NCopyVariant=Disabled  FilterICVariant=InternalICsFilter  IntegratorICVariant=InternalICs  ExternalResetVariant=Disabled  TRSumVariant=Passthrough  SumFdbkVariant=Disabled  SumVariant=Sum_PID  TsampFilterVariant=InternalTs  TsampNgainVariant=Passthrough  TsampIntegralVariant=Passthrough  ExternalSaturationOutDataTypeStr=Inherit: Same as second input  aMode=0
  PID_x : slpidlib/PID Controller  Controller=PID  Form=Parallel  TimeDomain=Discrete-time  UseExternalTs=off  SampleTime=-1  IntegratorMethod=Forward Euler  FilterMethod=Forward Euler  ControllerParametersSource=internal  P=0.85  I=0  UseKiTs=off  D=0  N=1  UseFilter=on  TunerSelectOption=Transfer Function Based (PID Tuner App)  InitialConditionSource=internal  InitialConditionForIntegrator=0  InitialConditionForFilter=0  DifferentiatorICPrevScaledInput=0  ExternalReset=none  TrackingMode=off  Kt=1  LimitOutput=on  SatLimitsSource=internal  UpperSaturationLimit=20  LowerSaturationLimit=-20  LinearizeAsGain=off  AntiWindupMode=none  Kb=1  POutMin=[]  POutMax=[]  IOutMin=[]  IOutMax=[]  DOutMin=[]  DOutMax=[]  NOutMin=[]  NOutMax=[]  SumOutMin=[]  SumOutMax=[]  SaturationOutMin=[]  SaturationOutMax=[]  PParamMin=[]  PParamMax=[]  IParamMin=[]  IParamMax=[]  DParamMin=[]  DParamMax=[]  NParamMin=[]  NParamMax=[]  KbParamMin=[]  KbParamMax=[]  KtParamMin=[]  KtParamMax=[]  KbOutMin=[]  KbOutMax=[]  KtOutMin=[]  KtOutMax=[]  IntegratorOutMin=[]  IntegratorOutMax=[]  FilterOutMin=[]  FilterOutMax=[]  SumI1OutMin=[]  SumI1OutMax=[]  SumI2OutMin=[]  SumI2OutMax=[]  SumI3OutMin=[]  SumI3OutMax=[]  SumI4OutMin=[]  SumI4OutMax=[]  SumDOutMin=[]  SumDOutMax=[]  DifferentiatorOutMin=[]  DifferentiatorOutMax=[]  FilterDiffOutCoefMin=[]  FilterDiffOutCoefMax=[]  ReciprocalOutMin=[]  ReciprocalOutMax=[]  SumDenOutMin=[]  SumDenOutMax=[]  SumNumOutMin=[]  SumNumOutMax=[]  DivideOutMin=[]  DivideOutMax=[]  UdiffTsProdOutMin=[]  UdiffTsProdOutMax=[]  NTsProdOutMin=[]  NTsProdOutMax=[]  UintegralTsProdOutMin=[]  UintegralTsProdOutMax=[]  UngainTsProdOutMin=[]  UngainTsProdOutMax=[]  IntegratorContinuousStateAttributes=''  IntegratorStateMustResolveToSignalObject=off  IntegratorRTWStateStorageClass=Auto  FilterContinuousStateAttributes=''  FilterStateMustResolveToSignalObject=off  FilterRTWStateStorageClass=Auto  ParallelPVariant=InternalParameters  IdealPVariant=Disabled  IVariant=InternalParameters  DVariant=InternalParameters  IntegratorVariant=Discrete  SatVariant=Enabled  AWVariant=Passthrough  PCopyVariant=Disabled  TRVariant=Disabled  FdbkBlocksVariant=Forward  IdealPFdbkVariant=Disabled  SatFdbkVariant=Disabled  DerivativeFilterVariant=ForwardEulerFilter  NVariant=InternalParameters  NCopyVariant=Disabled  FilterICVariant=InternalICsFilter  IntegratorICVariant=InternalICs  ExternalResetVariant=Disabled  TRSumVariant=Passthrough  SumFdbkVariant=Disabled  SumVariant=Sum_PID  TsampFilterVariant=InternalTs  TsampNgainVariant=Passthrough  TsampIntegralVariant=Passthrough  ExternalSaturationOutDataTypeStr=Inherit: Same as second input  aMode=0
  PID_y : slpidlib/PID Controller  Controller=PID  Form=Parallel  TimeDomain=Discrete-time  UseExternalTs=off  SampleTime=-1  IntegratorMethod=Backward Euler  FilterMethod=Forward Euler  ControllerParametersSource=internal  P=0.85  I=0  UseKiTs=off  D=0  N=1  UseFilter=on  TunerSelectOption=Transfer Function Based (PID Tuner App)  InitialConditionSource=internal  InitialConditionForIntegrator=0  InitialConditionForFilter=0  DifferentiatorICPrevScaledInput=0  ExternalReset=none  TrackingMode=off  Kt=1  LimitOutput=on  SatLimitsSource=internal  UpperSaturationLimit=20  LowerSaturationLimit=-20  LinearizeAsGain=off  AntiWindupMode=none  Kb=1  POutMin=[]  POutMax=[]  IOutMin=[]  IOutMax=[]  DOutMin=[]  DOutMax=[]  NOutMin=[]  NOutMax=[]  SumOutMin=[]  SumOutMax=[]  SaturationOutMin=[]  SaturationOutMax=[]  PParamMin=[]  PParamMax=[]  IParamMin=[]  IParamMax=[]  DParamMin=[]  DParamMax=[]  NParamMin=[]  NParamMax=[]  KbParamMin=[]  KbParamMax=[]  KtParamMin=[]  KtParamMax=[]  KbOutMin=[]  KbOutMax=[]  KtOutMin=[]  KtOutMax=[]  IntegratorOutMin=[]  IntegratorOutMax=[]  FilterOutMin=[]  FilterOutMax=[]  SumI1OutMin=[]  SumI1OutMax=[]  SumI2OutMin=[]  SumI2OutMax=[]  SumI3OutMin=[]  SumI3OutMax=[]  SumI4OutMin=[]  SumI4OutMax=[]  SumDOutMin=[]  SumDOutMax=[]  DifferentiatorOutMin=[]  DifferentiatorOutMax=[]  FilterDiffOutCoefMin=[]  FilterDiffOutCoefMax=[]  ReciprocalOutMin=[]  ReciprocalOutMax=[]  SumDenOutMin=[]  SumDenOutMax=[]  SumNumOutMin=[]  SumNumOutMax=[]  DivideOutMin=[]  DivideOutMax=[]  UdiffTsProdOutMin=[]  UdiffTsProdOutMax=[]  NTsProdOutMin=[]  NTsProdOutMax=[]  UintegralTsProdOutMin=[]  UintegralTsProdOutMax=[]  UngainTsProdOutMin=[]  UngainTsProdOutMax=[]  IntegratorContinuousStateAttributes=''  IntegratorStateMustResolveToSignalObject=off  IntegratorRTWStateStorageClass=Auto  FilterContinuousStateAttributes=''  FilterStateMustResolveToSignalObject=off  FilterRTWStateStorageClass=Auto  ParallelPVariant=InternalParameters  IdealPVariant=Disabled  IVariant=InternalParameters  DVariant=InternalParameters  IntegratorVariant=Discrete  SatVariant=Enabled  AWVariant=Passthrough  PCopyVariant=Disabled  TRVariant=Disabled  FdbkBlocksVariant=Forward  IdealPFdbkVariant=Disabled  SatFdbkVariant=Disabled  DerivativeFilterVariant=ForwardEulerFilter  NVariant=InternalParameters  NCopyVariant=Disabled  FilterICVariant=InternalICsFilter  IntegratorICVariant=InternalICs  ExternalResetVariant=Disabled  TRSumVariant=Passthrough  SumFdbkVariant=Disabled  SumVariant=Sum_PID  TsampFilterVariant=InternalTs  TsampNgainVariant=Passthrough  TsampIntegralVariant=Passthrough  ExternalSaturationOutDataTypeStr=Inherit: Same as second input  aMode=0
  "Rotation mat " : MATLAB Function  TreatAsAtomicUnit=on
  desire_pitch : Outport
  desire_roll : Outport  Port=2
  wires:
  x/1 -> PID_x/1
  y/1 -> PID_y/1
  [vx] -> Mux1/1  "vx"
  [vy] -> Mux1/2
  PID_x/1 -> Mux/1
  PID_y/1 -> Mux/2
  [Yaw] -> "Rotation mat "/1(yaw)
  Mux/1 -> Minus2/1
  Mux1/1 -> Minus2/2
  Minus2/1 -> Matrix Multiply/2
  "Rotation mat "/1(R) -> Matrix Multiply/1
  Matrix Multiply/1 -> Demux/1
  Demux/1 -> PID_vx/1
  Demux/2 -> PID_vy/1
  PID_vy/1 -> desire_roll/1
  PID_vx/1 -> desire_pitch/1

== matlab function No6_QuadcopterTrackPositionControl/Subsystem/Rotation mat  ==
  data: yaw input; R output
function R = get_r_mat(yaw)
R = [-cos(yaw) sin(yaw); sin(yaw) cos(yaw)]';

== stateflow chart No6_QuadcopterTrackPositionControl/Chart ==
  state Start_Up
    state Takeoff
      entry:
      t1=t;
      during:
      controlAltitude(1);
    state Ready
      entry,during:
      if Z < 1&& Z > -1
      state=1;
      end
    (default) -> Ready
    Ready -> (junction 87) : [Arm==1&&state==1]
    (junction 87) -> Takeoff [order 1] : [~AllControl]
  state controlAltitude(bool) [function]
    (default) -> (junction 51) : {Z_Control=bool;}
  state controlAttitude(bool) [function]
    (default) -> (junction 38) : {Attitude_Control=bool;}
  state Position_Control
    state Hold [parallel]
      entry,during:
      controlAltitude(1);
      settings: executionOrder=1
    state Attitude [parallel]
      entry,during:
      controlAttitude(1);
      settings: executionOrder=2
    state Position [parallel]
      entry,during:
      controlPosition(1);
      settings: executionOrder=3
  state controlPosition(bool) [function]
    (default) -> (junction 67) : {Position_Control=bool;}
  (default) -> Start_Up
  (junction 87) -> Position_Control [order 2] : [AllControl]
  Takeoff -> Position_Control : [E_z*sign(E_z)<0.3 &&t-t1>0.5]
  data: bool function_input; bool function_input; bool function_input; Arm input size=1; Z_Control output; Z input size=1; state local; E_z input size=1; Attitude_Control output; Position_Control output; i local; t input; t1 local; AllControl input

== matlab function No6_QuadcopterTrackPositionControl/x_d, y_d Generator ==
  data: x_d output; y_d output; t input; number input
function [x_d, y_d] = fcn(t,number)
%--------------------------------------------------------------------------
% Set Parameters:
%pi = 3.14159265358;
r=2;
T=20;
omega=2*pi/T;
t_f=T/4;
%--------------------------------------------------------------------------
% Define temp of outputs
o_X = 0;         o_Y = 0;
dot_o_X  = 0;    dot_o_Y  = 0;
%--------------------------------------------------------------------------
% Construct outputs:
n = number;
switch n
    case 1
        o_Y = r*sin(2*omega*t);
        o_X=2*r*sin(omega*t)*sin(omega*t);
        
    case 2
        o_X = 0;
        o_Y = 0;
end
%--------------------------------------------------------------------------
% Output:
x_d = o_X;

y_d = o_Y;

%--------------------------------------------------------------------------

== matlab function No6_QuadcopterTrackPositionControl/MATLAB Function2 ==
  data: qx input; qy input; phi_d output; qz input; psi_d input; theta_d output; u input
function [phi_d,theta_d] = fcn(qx,qy,qz,psi_d,u)
g = 9.8;
m =0.8;
c = m*(qx*sin(psi_d)-qy*cos(psi_d))/u;
if abs(c) <= 1
    a = asin(c);
else
    a = asin(abs(c)/c*1);
end
b = atan((qx*cos(psi_d)+qy*sin(psi_d))/(g+qz));
if a>pi/6
    a = pi/6;
elseif a<-pi/6
    a = -pi/6;   
end
if b>pi
    b = pi;
elseif b<-pi/6
    b = -pi/6;
end
phi_d = a;
theta_d = -b;
%Zhao B, Xian B, Zhang Y, et al. Nonlinear robust adaptive tracking control of a quadrotor UAV via immersion and invariance methodology[J]. IEEE Transactions on Industrial Electronics, 2014, 62(5): 2891-2902.

== matlab function No6_QuadcopterTrackPositionControl/MATLAB Function1 ==
  data: phi input; u output; theta input
function u = fcn(phi,theta)
m = 0.8;
g = 9.8;
u =m*g/(cos(theta)*cos(phi)) ;
